simulink model "motor_model_23b_nyquist"  (R2025b)
settings: Solver=VariableStepAuto  StartTime=0.0  StopTime=2  RelTol=1e-3
values from neighbouring files (symbols this model uses):
  D = 8.57e-7    (= 8.57e-07)    [motor_model_m.m]    (also in sampling_exercise.m)
  gear = 9.68    [motor_model_m.m]    (also in sampling_exercise.m = 9.6)
  J = 0.94e-6    (= 9.4e-07)    [motor_model_m.m]    (also in sampling_exercise.m)
  Kb = Kt    (= 0.008863)    [motor_model_m.m]    (also in sampling_exercise.m)
  Kp = 0.05    [sampling_exercise.m]
  Kt = 0.008863    [motor_model_m.m]    (also in sampling_exercise.m)
  L = 3.57e-3    (= 0.00357)    [motor_model_m.m]    (also in sampling_exercise.m)
  R = 3.57    [motor_model_m.m]    (also in sampling_exercise.m)
  r2m = wheelRadius/gear    (= 0.00309917355372)    [motor_model_m.m]    (also in sampling_exercise.m = 0.003125)
  Ts = 1    [lecture_4.m]    (also in sampling_exercise.m = Ts_values(i))
  wrad = 0.03    [sampling_exercise.m]
settings Model: Creator=chr  LastModifiedBy=User1

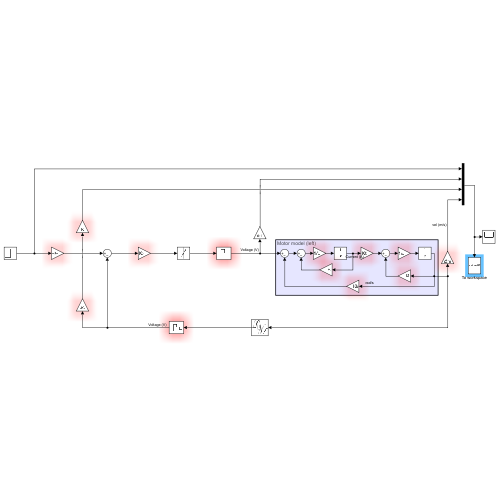
[thumbnail: Simulink's stored preview of the top-level diagram]
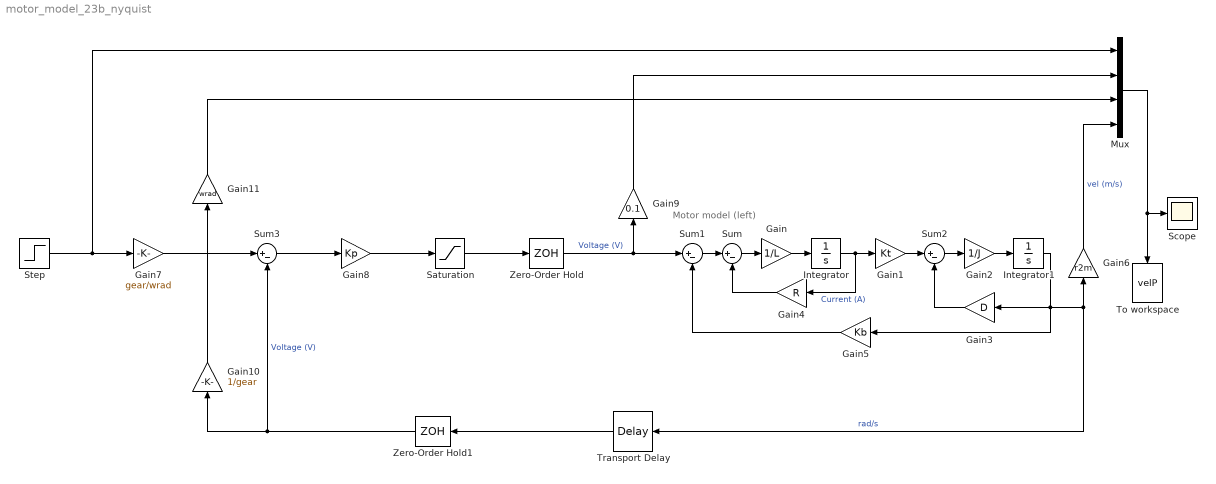
== system motor_model_23b_nyquist ==
  note: Motor model (left)
  Gain : Gain  Gain=1/L
  Gain1 : Gain  Gain=Kt
  Gain10 : Gain  Gain=1/gear
  Gain11 : Gain  Gain=wrad
  Gain2 : Gain  Gain=1/J
  Gain3 : Gain  Gain=D
  Gain4 : Gain  Gain=R
  Gain5 : Gain  Gain=Kb
  Gain6 : Gain  Gain=r2m
  Gain7 : Gain  Gain=gear/wrad
  Gain8 : Gain  Gain=Kp
  Gain9 : Gain  Gain=0.1
  Integrator : Integrator
  Integrator1 : Integrator
  Mux : Mux
  Saturation : Saturate  UpperLimit=9  LowerLimit=-9
  Scope : Scope
      settings: ActiveDisplayYMinimum=-0.28935  ActiveDisplayYMaximum=6.07084
  Step : Step  Time=0.2  After=0.1  SampleTime=0
  Sum{,1..3} (4 alike) : Sum  Inputs=|+-
  To workspace : ToWorkspace  VariableName=velP  SaveFormat=Timeseries  SampleTime=-1
  Transport Delay : TransportDelay  DelayTime=0.01
  Zero-Order Hold : ZeroOrderHold  SampleTime=Ts
  Zero-Order Hold1 : ZeroOrderHold  SampleTime=Ts
  wires:
  Gain/1 -> Integrator/1
  Sum/1 -> Gain/1
  Integrator/1 -> Gain4/1, Gain1/1  "Current (A)"
  Sum1/1 -> Sum/1
  Gain1/1 -> Sum2/1
  Sum2/1 -> Gain2/1
  Gain2/1 -> Integrator1/1
  Integrator1/1 -> Gain3/1, Gain5/1, Transport Delay/1, Gain6/1  "rad/s"
  Gain3/1 -> Sum2/2
  Gain4/1 -> Sum/2
  Gain5/1 -> Sum1/2
  Mux/1 -> Scope/1, To workspace/1
  Gain6/1 -> Mux/4  "vel (m/s)"
  Zero-Order Hold/1 -> Gain9/1, Sum1/1  "Voltage (V)"
  Step/1 -> Mux/1, Gain7/1
  Gain7/1 -> Sum3/1
  Sum3/1 -> Gain8/1
  Saturation/1 -> Zero-Order Hold/1
  Gain8/1 -> Saturation/1
  Transport Delay/1 -> Zero-Order Hold1/1
  Zero-Order Hold1/1 -> Gain10/1, Sum3/2  "Voltage (V)"
  Gain9/1 -> Mux/2
  Gain10/1 -> Gain11/1
  Gain11/1 -> Mux/3
